simulink model "LCK_DanishV01"  (R2018b)
settings: Solver=FixedStepDiscrete  StartTime=0.0  StopTime=inf  FixedStep=0.01  RelTol=1e-3
PostLoadFcn:
  | if any(exist('dsrtsu_mdlpostloadfcn', 'file') ~= 0), dsrtsu_mdlpostloadfcn('Execute', bdroot); end
values from neighbouring files (symbols this model uses):
  C_DEG2RAD = 0.0175    [LCK_Macro.sldd]
  C_KPH2MPS = 0.2778    [LCK_Macro.sldd]
  C_NEARZERO = 0.0001    [LCK_Macro.sldd]
  C_ONE = 1.0    [LCK_Macro.sldd]
  C_RAD2DEG = 57.2958    [LCK_Macro.sldd]
  C_ZERO = 0.0    [LCK_Macro.sldd]
  k_accel_pedal_pos_per_speed_x : value not decoded    [LCK_LogicPara.sldd]
  k_accel_pedal_pos_per_speed_z : value not decoded    [LCK_LogicPara.sldd]
  k_brake_suprress_hold = 1000.0    [LCK_LogicPara.sldd]
  k_driver_appl_torque_filt = 50.0    [LCK_LogicPara.sldd]
  k_driver_suppression_hold_time = 3000.0    [LCK_LogicPara.sldd]
  k_hands_on_wheel_hold_msec = 500.0    [LCK_LogicPara.sldd]
  k_hands_on_wheel_torque_hi = 0.2    [LCK_LogicPara.sldd]
  k_hands_on_wheel_torque_lo = 0.15    [LCK_LogicPara.sldd]
  k_handsoff_delay_cycles = 50.0    [LCK_LogicPara.sldd]
  k_handsoff_torq_Lo_CR = 0.3    [LCK_LogicPara.sldd]
  k_handson_delay_cycles = 5.0    [LCK_LogicPara.sldd]
  k_HighAccel_suppress_hold = 3000.0    [LCK_LogicPara.sldd]
  k_HLR_suprress_hold = 3000.0    [LCK_LogicPara.sldd]
  k_hs_StrAng_CR_threshold_z : value not decoded    [LCK_LogicPara.sldd]
  k_LC_Exit_Switch = 0.0    [LCK_LogicPara.sldd]
  k_LCG_Configured = 1.0    [LCK_LogicPara.sldd]
  k_LCK_A0_Rdy2Act_UseConst = 0.0    [LCK_LogicPara.sldd]
  k_LCK_A0Fac_ActSta : value not decoded    [LCK_CtrlPara.sldd]
  k_LCK_A0Fac_DrvStm : value not decoded    [LCK_CtrlPara.sldd]
  k_LCK_A0Shift_LftCurv : value not decoded    [LCK_CtrlPara.sldd]
  k_LCK_A0Shift_RgtCurv : value not decoded    [LCK_CtrlPara.sldd]
  k_LCK_A0Shift_StraLan = 0.0    [LCK_CtrlPara.sldd]
  k_LCK_A0ShiftFac_Dy_LftCurv : value not decoded    [LCK_CtrlPara.sldd]
  k_LCK_A0ShiftFac_Dy_RgtCurv : value not decoded    [LCK_CtrlPara.sldd]
  k_LCK_A0ShiftFac_Vspd : value not decoded    [LCK_CtrlPara.sldd]
  k_LCK_accel_inhibit_thold = 35.0    [LCK_LogicPara.sldd]
  k_LCK_Active2Ready_Mask = 255.0    [LCK_LogicPara.sldd]
  k_LCK_CvatRateBks : value not decoded    [LCK_CtrlPara.sldd]
  k_LCK_CvatrBks : value not decoded    [LCK_CtrlPara.sldd]
  k_LCK_DFac_Dy : value not decoded    [LCK_CtrlPara.sldd]
  k_LCK_DFac_Dy_Curv : value not decoded    [LCK_CtrlPara.sldd]
  k_LCK_DFac_HaCurCen : value not decoded    [LCK_CtrlPara.sldd]
  k_LCK_DFac_HaCurSid : value not decoded    [LCK_CtrlPara.sldd]
  k_LCK_DFac_HadCurCen : value not decoded    [LCK_CtrlPara.sldd]
  k_LCK_DFac_HadCurSid : value not decoded    [LCK_CtrlPara.sldd]
  k_LCK_DFac_HadStrCen : value not decoded    [LCK_CtrlPara.sldd]
  k_LCK_DFac_HadStrSid : value not decoded    [LCK_CtrlPara.sldd]
  k_LCK_DFac_HaStrCen : value not decoded    [LCK_CtrlPara.sldd]
  k_LCK_DFac_HaStrSid : value not decoded    [LCK_CtrlPara.sldd]
  k_LCK_DFac_Rad : value not decoded    [LCK_CtrlPara.sldd]
  k_LCK_DFac_SA_CurCen : value not decoded    [LCK_CtrlPara.sldd]
  k_LCK_DFac_SA_CurSid : value not decoded    [LCK_CtrlPara.sldd]
  k_LCK_DFac_SA_StrCen : value not decoded    [LCK_CtrlPara.sldd]
  k_LCK_DFac_SA_StrSid : value not decoded    [LCK_CtrlPara.sldd]
  k_LCK_DFac_SS_CurCen : value not decoded    [LCK_CtrlPara.sldd]
  k_LCK_DFac_SS_CurSid : value not decoded    [LCK_CtrlPara.sldd]
  k_LCK_DFac_SS_StrCen : value not decoded    [LCK_CtrlPara.sldd]
  k_LCK_DFac_SS_StrSid : value not decoded    [LCK_CtrlPara.sldd]
  k_LCK_DFac_Vspd : value not decoded    [LCK_CtrlPara.sldd]
  k_LCK_DlyTm_DrvStim = 0.2    [LCK_CtrlPara.sldd]
  k_LCK_DTermMax = 2.0    [LCK_CtrlPara.sldd]
  k_LCK_DyBks_Curv : value not decoded    [LCK_CtrlPara.sldd]
  k_LCK_Enable_POOnly = 1.0    [LCK_LogicPara.sldd]
  k_LCK_Entry_DistBuffer = 0.1    [LCK_LogicPara.sldd]
  k_LCK_Fac_Vspd2RngThr_FalRec = 0.23    [LCK_CtrlPara.sldd]
  k_LCK_Ffw_CvatSwh = 0.0    [LCK_CtrlPara.sldd]
  k_LCK_Ffw_DyBks : value not decoded    [LCK_CtrlPara.sldd]
  k_LCK_Ffw_TimCon_CmdFlt = 0.0    [LCK_CtrlPara.sldd]
  k_LCK_FfwDeltaFac_Rad_Lft : value not decoded    [LCK_CtrlPara.sldd]
  k_LCK_FfwDeltaFac_Rad_Rgt : value not decoded    [LCK_CtrlPara.sldd]
  k_LCK_FfwDeltaFac_Vspd : value not decoded    [LCK_CtrlPara.sldd]
  k_LCK_FfwFac_CvatRate_Lft : value not decoded    [LCK_CtrlPara.sldd]
  k_LCK_FfwFac_CvatRate_Rgt : value not decoded    [LCK_CtrlPara.sldd]
  k_LCK_FfwFac_Dy : value not decoded    [LCK_CtrlPara.sldd]
  k_LCK_FfwFac_Rad_Lft : value not decoded    [LCK_CtrlPara.sldd]
  k_LCK_FfwFac_Rad_Rgt : value not decoded    [LCK_CtrlPara.sldd]
  k_LCK_FfwFac_Vspd : value not decoded    [LCK_CtrlPara.sldd]
  k_LCK_FfwTorq_Cvat : value not decoded    [LCK_CtrlPara.sldd]
  k_LCK_HAFac_ActSta : value not decoded    [LCK_CtrlPara.sldd]
  k_LCK_HAFac_DrvStm : value not decoded    [LCK_CtrlPara.sldd]
  k_LCK_HaloTime = 2000.0    [LCK_LogicPara.sldd]
  k_LCK_HaloTime_Switch = 0.0    [LCK_LogicPara.sldd]
  k_LCK_HARFac_ActSta : value not decoded    [LCK_CtrlPara.sldd]
  k_LCK_HARFac_DrvStm : value not decoded    [LCK_CtrlPara.sldd]
  k_LCK_Hed_DyBks : value not decoded    [LCK_CtrlPara.sldd]
  k_LCK_HedAngDiffX : value not decoded    [LCK_CtrlPara.sldd]
  k_LCK_HedAngRateDiffX : value not decoded    [LCK_CtrlPara.sldd]
  k_LCK_HndsOnWhel_DlyTm_Idl2Rdy = 0.0    [LCK_LogicPara.sldd]
  k_LCK_host_veh_width = 1.86    [LCK_LogicPara.sldd]
  k_LCK_Idle2Ready_Mask = 239.0    [LCK_LogicPara.sldd]
  k_LCK_Junc_SusTime = 1.0    [LCK_LogicPara.sldd]
  k_LCK_KpKdDecSlopeLmt = 10.0    [LCK_CtrlPara.sldd]
  k_LCK_KpKdIncSlopeLmt = 5.0    [LCK_CtrlPara.sldd]
  k_LCK_Lat_Ctrl_DFac_Lft = 1.0    [LCK_CtrlPara.sldd]
  k_LCK_Lat_Ctrl_DFac_Rgt = 1.05    [LCK_CtrlPara.sldd]
  k_LCK_Lat_Ctrl_Kd = 0.8    [LCK_CtrlPara.sldd]
  k_LCK_Lat_Ctrl_Ki = 0.5    [LCK_CtrlPara.sldd]
  k_LCK_Lat_Ctrl_Kp = 0.7    [LCK_CtrlPara.sldd]
  k_LCK_Lat_Ctrl_Kp_NearGain = 0.7    [LCK_CtrlPara.sldd]
  k_LCK_Lat_Ctrl_PFac_Lft = 1.0    [LCK_CtrlPara.sldd]
  k_LCK_Lat_Ctrl_PFac_Rgt = 1.05    [LCK_CtrlPara.sldd]
  k_LCK_Lat_Ctrl_TimCon_CmdFlt = 5.0    [LCK_CtrlPara.sldd]
  k_LCK_Lat_DFac_Rad : value not decoded    [LCK_CtrlPara.sldd]
  k_LCK_Lat_DFac_SS_Cur : value not decoded    [LCK_CtrlPara.sldd]
  k_LCK_Lat_DFac_SS_Str : value not decoded    [LCK_CtrlPara.sldd]
  k_LCK_Lat_DFac_Vspd : value not decoded    [LCK_CtrlPara.sldd]
  k_LCK_Lat_DyBks : value not decoded    [LCK_CtrlPara.sldd]
  k_LCK_Lat_IFac_Rad : value not decoded    [LCK_CtrlPara.sldd]
  k_LCK_Lat_IFac_Vspd : value not decoded    [LCK_CtrlPara.sldd]
  k_LCK_Lat_ILmtFac_Dy_CurvLan : value not decoded    [LCK_CtrlPara.sldd]
  k_LCK_Lat_ILmtFac_Dy_StraLan : value not decoded    [LCK_CtrlPara.sldd]
  k_LCK_Lat_ILmtFac_Rad : value not decoded    [LCK_CtrlPara.sldd]
  k_LCK_Lat_ILmtFac_Rad_NearGain = 1.0    [LCK_CtrlPara.sldd]
  k_LCK_Lat_ILmtFac_Vspd_CurvLan : value not decoded    [LCK_CtrlPara.sldd]
  k_LCK_Lat_ILmtFac_Vspd_StraLan : value not decoded    [LCK_CtrlPara.sldd]
  k_LCK_Lat_ITermLmt_Dy = 1.0    [LCK_CtrlPara.sldd]
  k_LCK_Lat_KpKdDecSlopeLmt = 10.0    [LCK_CtrlPara.sldd]
  k_LCK_Lat_KpKdIncSlopeLmt = 10.0    [LCK_CtrlPara.sldd]
  k_LCK_Lat_PFac_Dy_InnLftCur : value not decoded    [LCK_CtrlPara.sldd]
  k_LCK_Lat_PFac_Dy_InnRgtCur : value not decoded    [LCK_CtrlPara.sldd]
  k_LCK_Lat_PFac_Dy_OutLftCur : value not decoded    [LCK_CtrlPara.sldd]
  k_LCK_Lat_PFac_Dy_OutRgtCur : value not decoded    [LCK_CtrlPara.sldd]
  k_LCK_Lat_PFac_Dy_Str : value not decoded    [LCK_CtrlPara.sldd]
  k_LCK_Lat_PFac_Rad : value not decoded    [LCK_CtrlPara.sldd]
  ... (+153 more)
undefined symbols (not defined in the file or in its folder): k_LCK_CurvBks, K_LCK_SPA0A1A2_LMRngCmp_y
libraries: LateralControl_fcns_lib x58, simulink x24
(part 10 of 47)

== system LCK_DanishV01/Lateral_Control_Module/Adas_Lateral_Control_LCK_Core/Module 6 ==
  Road_Radius : Inport
  Curvature_0 : Inport  Port=2
  Dy_1 : Inport  Port=3
  Dy_0 : Inport  Port=4
  Determination Of Cen Flag : Subsystem
  Determination of Str Flag : Subsystem
  Recognition of Curve Information : Subsystem
  Str_Flag : Outport
  Cen_Flag : Outport  Port=2
  Inn_Cur_Flag_1 : Outport  Port=3
  Inn_Cur_Flag_0 : Outport  Port=4
  Cur_Lan_Flag : Outport  Port=5
  wires:
  Dy_1/1 -> Recognition of Curve Information/2(Dy_1)
  Road_Radius/1 -> Determination of Str Flag/1(Road_Radius)
  Determination Of Cen Flag/1(Cen_Flag) -> Cen_Flag/1
  Recognition of Curve Information/3(Cur_Lan_Flag) -> Cur_Lan_Flag/1
  Recognition of Curve Information/2(Inn_Cur_Flag_0) -> Inn_Cur_Flag_0/1
  Recognition of Curve Information/1(Inn_Cur_Flag_1) -> Inn_Cur_Flag_1/1
  Curvature_0/1 -> Recognition of Curve Information/3(Curvature_0)
  Dy_0/1 -> Determination Of Cen Flag/2(Dy_0), Recognition of Curve Information/1(Dy_0)
  Determination of Str Flag/1(Str_Flag) -> Str_Flag/1, Determination Of Cen Flag/1(Str_Flag)

== system LCK_DanishV01/Lateral_Control_Module/Adas_Lateral_Control_LCK_Core/Module 7 ==
  Signal_Weakened_Flag : Inport
  Lat_Ctrl_State : Inport  Port=2
  Bus Selector8 : BusSelector  OutputSignals=Act_Start_Falg_Held,Drv_Stm_Flag_Held
  Compare To Constant4 : simulink/Logic and Bit Operations/Compare To Constant  relop===  const=0  OutDataTypeStr=boolean
  Constant : Constant  Value=0  OutDataTypeStr=boolean
  Logical Operator : Logic  Operator=OR  Inputs=3  AllPortsSameDT=off  OutDataTypeStr=boolean
  I_Term_Reset_Flag : Outport
  I_Term_Frozen_Flag : Outport  Port=2
  wires:
  Lat_Ctrl_State/1 -> Compare To Constant4/1
  Signal_Weakened_Flag/1 -> Bus Selector8/1
  Bus Selector8/1 -> Logical Operator/1  "<Act_Start_Falg_Held>"
  Bus Selector8/2 -> Logical Operator/2  "<Drv_Stm_Flag_Held>"
  Compare To Constant4/1 -> Logical Operator/3
  Logical Operator/1 -> I_Term_Reset_Flag/1
  Constant/1 -> I_Term_Frozen_Flag/1

== system LCK_DanishV01/Lateral_Control_Module/Adas_Lateral_Control_LCK_Core/Module 8 ==
  Vspd : Inport
  Dy_1 : Inport  Port=2
  Dy_0 : Inport  Port=3
  Lat_Rate : Inport  Port=4
  Road_Radius : Inport  Port=5
  Steer_Spd : Inport  Port=6
  PosLan_Info : Inport  Port=7
  I_Term_CtrlState : Inport  Port=8
  Bus Creator : BusCreator  Inputs=8
  Bus Selector1 : BusSelector  OutputSignals=I_Term_Reset_Flag,I_Term_Frozen_Flag
  Module 0 : Subsystem
  Module 1 : Subsystem
  Lat_Ctrl_Info : Outport
  wires:
  Module 0/1(P_Gain) -> Module 1/4(P_Gain)
  Module 0/2(I_Gain) -> Module 1/5(I_Gain)
  Module 0/3(D_Gain) -> Module 1/6(D_Gain)
  Module 0/4(ITerm_Limit) -> Module 1/7(ITerm_Limit)
  Dy_1/1 -> Module 0/1(Dy_1), Module 1/1(Dy_1)
  Lat_Rate/1 -> Module 0/3(Lat_Rate), Module 1/3(Lat_Rate)
  Dy_0/1 -> Module 0/2(Dy_0), Module 1/2(Dy_0)
  Vspd/1 -> Module 0/4(Vspd)
  Road_Radius/1 -> Module 0/5(Road_Radius)
  PosLan_Info/1 -> Module 0/7(PosLan_Info)
  Steer_Spd/1 -> Module 0/6(Steer_Spd)
  Bus Selector1/1 -> Module 1/8(LatCtrl_I_Reset_Flag)  "<I_Term_Reset_Flag>"
  Bus Selector1/2 -> Module 1/9(LatCtrl_ITerm_Frozen_Flag)  "<I_Term_Frozen_Flag>"
  I_Term_CtrlState/1 -> Bus Selector1/1
  Module 1/1(LatCtrl_Cmd) -> Bus Creator/1  "Lat_Ctr_Cmd"
  Module 1/2(LatCtrl_P_Term) -> Bus Creator/2  "Lat_Ctrl_PTerm"
  Module 1/3(LatCtrl_I_Term) -> Bus Creator/3  "Lat_Ctrl_ITerm"
  Module 1/4(LatCtrl_D_Term) -> Bus Creator/4  "Lat_Ctrl_DTerm"
  Module 1/5(LatCtrl_P_Term_0) -> Bus Creator/5  "Lat_Ctrl_PTerm_0"
  Module 1/6(LatCtrl_P_Term_1) -> Bus Creator/6  "Lat_Ctrl_PTerm_1"
  Module 1/7(LatCtrl_I_Term_0) -> Bus Creator/7  "Lat_Ctrl_ITerm_0"
  Module 1/8(LatOffsetCtrl_I_Term_1) -> Bus Creator/8  "Lat_Ctrl_ITerm_1"
  Bus Creator/1 -> Lat_Ctrl_Info/1

== system LCK_DanishV01/Lateral_Control_Module/Adas_Lateral_Control_LCK_Core/Module 9 ==
  Vspd : Inport
  Dy_0 : Inport  Port=2
  Hed_Ang : Inport  Port=3
  Hed_Ang_Rat : Inport  Port=4
  Steer_Ang : Inport  Port=5
  Steer_Spd : Inport  Port=6
  Road_Radius : Inport  Port=7
  Str_Flag : Inport  Port=8
  Cen_Flag : Inport  Port=9
  Bus Creator : BusCreator  Inputs=5
  Module 0 : Subsystem
  Module 1 : Subsystem
  LatCtrl_Info : Outport
  wires:
  Dy_0/1 -> Module 0/3(Dy_0)
  Hed_Ang/1 -> Module 0/1(Hed_Ang), Module 1/1(Hed_Ang)
  Str_Flag/1 -> Module 0/4(Str_Flag)
  Vspd/1 -> Module 0/5(Vspd)
  Road_Radius/1 -> Module 0/6(Road_Radius)
  Steer_Spd/1 -> Module 0/8(Steer_Spd)
  Hed_Ang_Rat/1 -> Module 1/2(Hed_Ang_Rat), Module 0/2(Hed_Ang_Diff_Rat)
  Module 1/1(LatCtrl_Cmd) -> Bus Creator/1  "LatCtrl_Cmd"
  Cen_Flag/1 -> Module 0/9(Cen_Flag)
  Bus Creator/1 -> LatCtrl_Info/1
  Steer_Ang/1 -> Module 0/7(Steer_Ang)
  Module 0/1(P_Gain) -> Bus Creator/4, Module 1/3(P_Gain)  "LatCtrl_P"
  Module 0/2(D_Gain) -> Bus Creator/5, Module 1/4(D_Gain)  "LatCtrl_D"
  Module 1/2(LatCtrl_P_Term) -> Bus Creator/2  "LatCtrl_PTerm"
  Module 1/3(LatCtrl_D_Term) -> Bus Creator/3  "LatCtrl_DTerm"

== system LCK_DanishV01/Lateral_Control_Module/Adas_Lateral_Control_LCK_Core/Process of SPP False Recognition ==
  LatCtrl_LCK_LanSigInputs : Inport
  LatCtrl_LCK_TrackSigInputs : Inport  Description=_GWMAB30P4.LCK.000_220_  Port=2
  Vspd : Inport  Port=3
  Bus Selector20 : BusSelector  OutputSignals=CIPV1ObjRange,CIPV1ObjTrackID
  Bus Selector21 : BusSelector  OutputSignals=VID_Lin_01_Range,VID_Lin_02_Range
  Constant10 : Constant  Value=0  OutDataTypeStr=uint8
  Constant2 : Constant  Value=4  OutDataTypeStr=uint8
  Constant5 : Constant  Value=0  OutDataTypeStr=uint8
  Constant6 : Constant  Value=2  OutDataTypeStr=uint8
  Constant8 : Constant  Value=2  OutDataTypeStr=uint8
  Constant9 : Constant  Value=3  OutDataTypeStr=uint8
  Divide1 : Product  Description=_GWMAB30P3.LCK.000_157_  Inputs=*/  OutDataTypeStr=single
  Product6 : Product
  Relational Operator : RelationalOperator  OutDataTypeStr=boolean  RndMeth=Nearest
  Relational Operator1 : RelationalOperator  Operator=>  OutDataTypeStr=boolean  RndMeth=Nearest
  Relational Operator2 : RelationalOperator  Operator=<  OutDataTypeStr=boolean  RndMeth=Nearest
  Sum3 : Sum  Description=_GWMAB30P2.LCK.000_1362_
  Switch1 : Switch  Description=_GWMAB30P2.LCK.000_1368_  Threshold=0.5  OutDataTypeStr=uint8
  Switch10 : Switch  Description=_GWMAB30P2.LCK.000_1368_  Threshold=0.5
  Switch8 : Switch  Description=_GWMAB30P2.LCK.000_1368_  Threshold=0.5  OutDataTypeStr=uint8
  k_LCK_Fac_Vspd2RngThr_FalRec : Constant  Value=k_LCK_Fac_Vspd2RngThr_FalRec
  k_LCK_RngThr_FalRec : Lookup_n-D  NumberOfTableDimensions=1  BreakpointsForDimension1=k_LCK_VspdBks  Table=k_LCK_RngThr_FalRec  ExtrapMethod=Clip  InternalRulePriority=Speed  RndMeth=Simplest  InputSameDT=on
  SPP_Recognition_Type : Outport
  wires:
  LatCtrl_LCK_LanSigInputs/1 -> Bus Selector21/1
  LatCtrl_LCK_TrackSigInputs/1 -> Bus Selector20/1
  Constant5/1 -> Relational Operator1/2
  Relational Operator2/1 -> Switch10/2
  k_LCK_Fac_Vspd2RngThr_FalRec/1 -> Product6/1
  Constant9/1 -> Switch10/3
  Constant10/1 -> Switch8/3
  Switch8/1 -> SPP_Recognition_Type/1
  Constant6/1 -> Divide1/2
  Constant8/1 -> Switch10/1
  Relational Operator/1 -> Switch8/2
  Relational Operator1/1 -> Switch1/2
  Constant2/1 -> Switch1/3
  Switch10/1 -> Switch1/1
  Switch1/1 -> Switch8/1
  Bus Selector20/2 -> Relational Operator1/1  "<CIPV1ObjTrackID>"
  Product6/1 -> Relational Operator2/1
  Bus Selector20/1 -> Relational Operator2/2  "<CIPV1ObjRange>"
  Vspd/1 -> Product6/2, k_LCK_RngThr_FalRec/1
  k_LCK_RngThr_FalRec/1 -> Relational Operator/1
  Bus Selector21/1 -> Sum3/1  "<VID_Lin_01_Range>"
  Bus Selector21/2 -> Sum3/2  "<VID_Lin_02_Range>"
  Sum3/1 -> Divide1/1
  Divide1/1 -> Relational Operator/2
